simulink library "LIB_TF_G_12_StepControl"  (Simulink 8.6)
settings: Solver=ode45  StartTime=0.0  StopTime=10.0  RelTol=1e-3
PreLoadFcn:
  | if exist('tl_preloadfcn','file'), tl_preloadfcn(gcs,402); end
PostLoadFcn:
  | if exist('tl_postloadfcn','file'), tl_postloadfcn(gcs,402); end
undefined symbols (not defined in the file): ddv, u2, u3
libraries: tllib x4, LIB_TF_G_12_StepControl x1
(part 6 of 7)

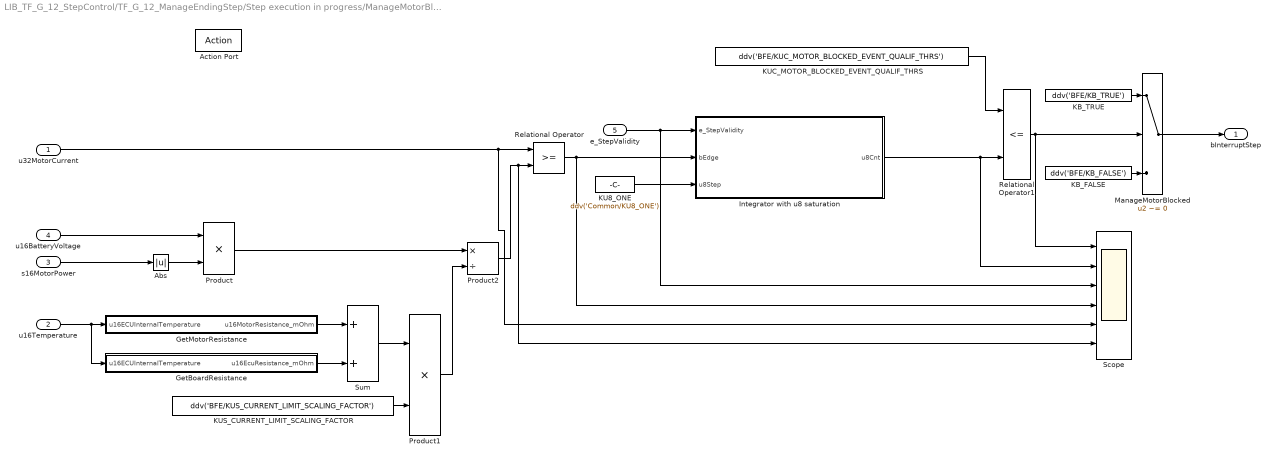
== system LIB_TF_G_12_StepControl/TF_G_12_ManageEndingStep/Step execution in progress/ManageMotorBlocked (Motor OverCurrent)/Motor Blocked Opt Activated/If Action Subsystem1 ==
  u32MotorCurrent : Inport  RequirementInfo={} %GIDa_b15262d0_e742_4384_8f9e_89978bbdea4b
  u16Temperature : Inport  RequirementInfo={} %GIDa_ef5c7aa1_d6d2_4676_bb67_ebadbb8854d8  Port=2
  s16MotorPower : Inport  RequirementInfo={} %GIDa_a7c6093a_f3fd_45c6_94cd_8623c3d3488b  Port=3
  u16BatteryVoltage : Inport  RequirementInfo={} %GIDa_ce521116_7135_4151_b5d9_8882b70060be  Port=4
  e_StepValidity : Inport  RequirementInfo={} %GIDa_ddfb933f_dae9_4570_b46d_68e419ca580a  Port=5
  Action Port : ActionPort  RequirementInfo={} %GIDa_51377548_8670_413b_8799_ae36625b9d74
  Abs : Abs  RequirementInfo={} %GIDa_8232010f_f8c2_4ccb_bbd6_00c9bee563e0  OutDataTypeStr=uint16  SaturateOnIntegerOverflow=on  mask(TL_Abs){data={'output',{'type','UInt16'},'date',735951.66847012728}}
      settings: CopyFcn=if exist('tl_reset_reviewflag','file')==2,tl_reset_reviewflag(gcbh);end  DeleteFcn=if exist('delete_tlblock','file')==2,delete_tlblock(gcbh);end  NameChangeFcn=if exist('rename_tlblock','file')==2,rename_tlblock(gcbh);end  OpenFcn=if exist('tl_open_blockdlg','file')==2,tl_open_blockdlg(gcbh);else,open_system(gcbh,'parameter');end
      mask Help: eval(['if exist(''tl_online_help'',''file'') == 2, tl_online_help(''Topic'',''TL_Abs''),else, web([''jar:file:///'',matlabroot,''/help/toolbox/simulink/help.jar!/slref/' lower(get_param(gcbh,'Blocktype')) '.html''], ''-helpbrowser''),end'])
      mask Display: plot([-0.05, 1.05, NaN, -0.05, 1.05],[.01, .01, NaN, .99, .99])
  GetBoardResistance : Subsystem  RequirementInfo={} %GIDa_d4bba72b_0433_4a1a_802a_6d5e3419819e  TreatAsAtomicUnit=on
  GetMotorResistance : Subsystem  RequirementInfo={} %GIDa_a7d90a02_c6c7_4e5e_b3b2_57b3a781c45c  TreatAsAtomicUnit=on
  Integrator with u8 saturation : Subsystem  RequirementInfo={} %GIDa_ba181890_6141_4dc0_bd10_b853b6348a4b  TreatAsAtomicUnit=on
  KB_FALSE : Constant  RequirementInfo={} %GIDa_a55cecaf_6f72_42fc_8a95_f0d92f6d4486  Value=ddv('BFE/KB_FALSE')  OutDataTypeStr=boolean  SampleTime=-1  mask(TL_Constant){data={'output',{'variable','BFE/KB_FALSE'},'date',735951.66846314818}}
      settings: CopyFcn=if exist('tl_reset_reviewflag','file')==2,tl_reset_reviewflag(gcbh);end  DeleteFcn=if exist('delete_tlblock','file')==2,delete_tlblock(gcbh);end  NameChangeFcn=if exist('rename_tlblock','file')==2,rename_tlblock(gcbh);end  OpenFcn=if exist('tl_open_blockdlg','file')==2,tl_open_blockdlg(gcbh);else,open_system(gcbh,'parameter');end
      mask Help: eval(['if exist(''tl_online_help'',''file'') == 2, tl_online_help(''Topic'',''TL_Constant''),else, web([''jar:file:///'',matlabroot,''/help/toolbox/simulink/help.jar!/slref/' lower(get_param(gcbh,'Blocktype')) '.html''], ''-helpbrowser''),end'])
      mask Display: plot([-0.05, 1.05, NaN, -0.05, 1.05],[.01, .01, NaN, .99, .99])
  KB_TRUE : Constant  RequirementInfo={} %GIDa_37d21bda_b46f_433f_b999_e144736c21a8  Value=ddv('BFE/KB_TRUE')  OutDataTypeStr=boolean  SampleTime=-1  mask(TL_Constant){data={'output',{'variable','BFE/KB_TRUE'},'date',735951.66846276622}}
      settings: CopyFcn=if exist('tl_reset_reviewflag','file')==2,tl_reset_reviewflag(gcbh);end  DeleteFcn=if exist('delete_tlblock','file')==2,delete_tlblock(gcbh);end  NameChangeFcn=if exist('rename_tlblock','file')==2,rename_tlblock(gcbh);end  OpenFcn=if exist('tl_open_blockdlg','file')==2,tl_open_blockdlg(gcbh);else,open_system(gcbh,'parameter');end
      mask Help: eval(['if exist(''tl_online_help'',''file'') == 2, tl_online_help(''Topic'',''TL_Constant''),else, web([''jar:file:///'',matlabroot,''/help/toolbox/simulink/help.jar!/slref/' lower(get_param(gcbh,'Blocktype')) '.html''], ''-helpbrowser''),end'])
      mask Display: plot([-0.05, 1.05, NaN, -0.05, 1.05],[.01, .01, NaN, .99, .99])
  KU8_ONE : Constant  RequirementInfo={} %GIDa_69ee802a_b870_416b_ab62_c046b6291559  Value=ddv('Common/KU8_ONE')  OutDataTypeStr=uint8  SampleTime=-1  mask(TL_Constant){data={'output',{'variable','Common/KU8_ONE'},'date',735951.66846239578}}
      settings: CopyFcn=if exist('tl_reset_reviewflag','file')==2,tl_reset_reviewflag(gcbh);end  DeleteFcn=if exist('delete_tlblock','file')==2,delete_tlblock(gcbh);end  NameChangeFcn=if exist('rename_tlblock','file')==2,rename_tlblock(gcbh);end  OpenFcn=if exist('tl_open_blockdlg','file')==2,tl_open_blockdlg(gcbh);else,open_system(gcbh,'parameter');end
      mask Help: eval(['if exist(''tl_online_help'',''file'') == 2, tl_online_help(''Topic'',''TL_Constant''),else, web([''jar:file:///'',matlabroot,''/help/toolbox/simulink/help.jar!/slref/' lower(get_param(gcbh,'Blocktype')) '.html''], ''-helpbrowser''),end'])
      mask Display: plot([-0.05, 1.05, NaN, -0.05, 1.05],[.01, .01, NaN, .99, .99])
  KUC_MOTOR_BLOCKED_EVENT_QUALIF_THRS : Constant  RequirementInfo={} %GIDa_b638c9ca_7e5c_4169_b0e7_1030e65cb8bd  Value=ddv('BFE/KUC_MOTOR_BLOCKED_EVENT_QUALIF_THRS')  OutDataTypeStr=uint8  SampleTime=-1  mask(TL_Constant){data={'output',{'variable','BFE/KUC_MOTOR_BLOCKED_EVENT_QUALIF_THRS'},'date',736308.64848615741}}
      settings: CopyFcn=if exist('tl_reset_reviewflag','file')==2,tl_reset_reviewflag(gcbh);end  DeleteFcn=if exist('delete_tlblock','file')==2,delete_tlblock(gcbh);end  NameChangeFcn=if exist('rename_tlblock','file')==2,rename_tlblock(gcbh);end  OpenFcn=if exist('tl_open_blockdlg','file')==2,tl_open_blockdlg(gcbh);else,open_system(gcbh,'parameter');end
      mask Help: eval(['if exist(''tl_online_help'',''file'') == 2, tl_online_help(''Topic'',''TL_Constant''),else, web([''jar:file:///'',matlabroot,''/help/toolbox/simulink/help.jar!/slref/' lower(get_param(gcbh,'Blocktype')) '.html''], ''-helpbrowser''),end'])
      mask Display: plot([-0.05, 1.05, NaN, -0.05, 1.05],[.01, .01, NaN, .99, .99])
  KUS_CURRENT_LIMIT_SCALING_FACTOR : Constant  RequirementInfo={} %GIDa_2f1f04c3_5d00_4e34_bf38_99862e862b9f  Value=ddv('BFE/KUS_CURRENT_LIMIT_SCALING_FACTOR')  OutDataTypeStr=uint16  SampleTime=-1  mask(TL_Constant){data={'output',{'variable','BFE/KUS_CURRENT_LIMIT_SCALING_FACTOR'},'date',735951.66846165515}}
      settings: CopyFcn=if exist('tl_reset_reviewflag','file')==2,tl_reset_reviewflag(gcbh);end  DeleteFcn=if exist('delete_tlblock','file')==2,delete_tlblock(gcbh);end  NameChangeFcn=if exist('rename_tlblock','file')==2,rename_tlblock(gcbh);end  OpenFcn=if exist('tl_open_blockdlg','file')==2,tl_open_blockdlg(gcbh);else,open_system(gcbh,'parameter');end
      mask Help: eval(['if exist(''tl_online_help'',''file'') == 2, tl_online_help(''Topic'',''TL_Constant''),else, web([''jar:file:///'',matlabroot,''/help/toolbox/simulink/help.jar!/slref/' lower(get_param(gcbh,'Blocktype')) '.html''], ''-helpbrowser''),end'])
      mask Display: plot([-0.05, 1.05, NaN, -0.05, 1.05],[.01, .01, NaN, .99, .99])
  ManageMotorBlocked : Switch  RequirementInfo={} %GIDa_9a329e77_4b29_4519_b45e_e6ed1365234e  Criteria=u2 ~= 0  mask(TL_Switch){data={'output',{'type','Bool'},'threshold',{'scalar',1},'date',735951.66846123838}}
      settings: CopyFcn=if exist('tl_reset_reviewflag','file')==2,tl_reset_reviewflag(gcbh);end  DeleteFcn=if exist('delete_tlblock','file')==2,delete_tlblock(gcbh);end  NameChangeFcn=if exist('rename_tlblock','file')==2,rename_tlblock(gcbh);end  OpenFcn=if exist('tl_open_blockdlg','file')==2,tl_open_blockdlg(gcbh);else,open_system(gcbh,'parameter');end
      mask Help: eval(['if exist(''tl_online_help'',''file'') == 2, tl_online_help(''Topic'',''TL_Switch''),else, web([''jar:file:///'',matlabroot,''/help/toolbox/simulink/help.jar!/slref/' lower(get_param(gcbh,'Blocktype')) '.html''], ''-helpbrowser''),end'])
      mask Display: plot([-0.05, 1.05, NaN, -0.05, 1.05],[.01, .01, NaN, .99, .99])
  Product : Product  RequirementInfo={} %GIDa_e4deacdf_ad83_4690_b51a_09e6e1684bb8  Inputs=**  OutDataTypeStr=uint32  RndMeth=Zero  mask(TL_Product){data={'output',{'type','UInt32'},'date',735951.66846074071}}
      settings: CopyFcn=if exist('tl_reset_reviewflag','file')==2,tl_reset_reviewflag(gcbh);end  DeleteFcn=if exist('delete_tlblock','file')==2,delete_tlblock(gcbh);end  NameChangeFcn=if exist('rename_tlblock','file')==2,rename_tlblock(gcbh);end  OpenFcn=if exist('tl_open_blockdlg','file')==2,tl_open_blockdlg(gcbh);else,open_system(gcbh,'parameter');end
      mask Help: eval(['if exist(''tl_online_help'',''file'') == 2, tl_online_help(''Topic'',''TL_Product''),else, web([''jar:file:///'',matlabroot,''/help/toolbox/simulink/help.jar!/slref/' lower(get_param(gcbh,'Blocktype')) '.html''], ''-helpbrowser''),end'])
      mask Display: plot([-0.05, 1.05, NaN, -0.05, 1.05],[.01, .01, NaN, .99, .99])
  Product1 : Product  RequirementInfo={} %GIDa_f39456aa_0ea8_4713_8ffb_570a378b51f3  Inputs=**  OutDataTypeStr=uint32  RndMeth=Zero  mask(TL_Product){data={'output',{'type','UInt32'},'date',735951.66846037039}}
      settings: CopyFcn=if exist('tl_reset_reviewflag','file')==2,tl_reset_reviewflag(gcbh);end  DeleteFcn=if exist('delete_tlblock','file')==2,delete_tlblock(gcbh);end  NameChangeFcn=if exist('rename_tlblock','file')==2,rename_tlblock(gcbh);end  OpenFcn=if exist('tl_open_blockdlg','file')==2,tl_open_blockdlg(gcbh);else,open_system(gcbh,'parameter');end
      mask Help: eval(['if exist(''tl_online_help'',''file'') == 2, tl_online_help(''Topic'',''TL_Product''),else, web([''jar:file:///'',matlabroot,''/help/toolbox/simulink/help.jar!/slref/' lower(get_param(gcbh,'Blocktype')) '.html''], ''-helpbrowser''),end'])
      mask Display: plot([-0.05, 1.05, NaN, -0.05, 1.05],[.01, .01, NaN, .99, .99])
  Product2 : Product  RequirementInfo={} %GIDa_a78a8f98_bcd9_4378_bd14_54184bd20a38  Inputs=*/  OutDataTypeStr=uint32  RndMeth=Zero  mask(TL_Product){data={'output',{'name','u32MaxCurrentThrs','type','UInt32'},'date',735951.66846}}
      settings: CopyFcn=if exist('tl_reset_reviewflag','file')==2,tl_reset_reviewflag(gcbh);end  DeleteFcn=if exist('delete_tlblock','file')==2,delete_tlblock(gcbh);end  NameChangeFcn=if exist('rename_tlblock','file')==2,rename_tlblock(gcbh);end  OpenFcn=if exist('tl_open_blockdlg','file')==2,tl_open_blockdlg(gcbh);else,open_system(gcbh,'parameter');end
      mask Help: eval(['if exist(''tl_online_help'',''file'') == 2, tl_online_help(''Topic'',''TL_Product''),else, web([''jar:file:///'',matlabroot,''/help/toolbox/simulink/help.jar!/slref/' lower(get_param(gcbh,'Blocktype')) '.html''], ''-helpbrowser''),end'])
      mask Display: plot([-0.05, 1.05, NaN, -0.05, 1.05],[.01, .01, NaN, .99, .99])
  Relational Operator : RelationalOperator  RequirementInfo={} %GIDa_ce1273a7_07a3_4d52_9644_bfe8f4081c88  OutDataTypeStr=boolean  mask(TL_RelationalOperator){data={'output',{'name','bMotorBlockedOccurence'},'date',735951.66845964117}}
      settings: DeleteFcn=if exist('delete_tlblock','file')==2,delete_tlblock(gcbh);end  NameChangeFcn=if exist('rename_tlblock','file')==2,rename_tlblock(gcbh);end  OpenFcn=if exist('tl_open_blockdlg','file')==2,tl_open_blockdlg(gcbh);else,open_system(gcbh,'parameter');end
      mask Help: eval(['if exist(''tl_online_help'',''file'') == 2, tl_online_help(''Topic'',''TL_RelationalOperator''),else, web([''jar:file:///'',matlabroot,''/help/toolbox/simulink/help.jar!/slref/' lower(get_param(gcbh,'Blocktype')) '.html''], ''-helpbrowser''),end'])
      mask Display: plot([-0.05, 1.05, NaN, -0.05, 1.05],[.01, .01, NaN, .99, .99])
  Relational Operator1 : RelationalOperator  RequirementInfo={} %GIDa_80bd2eb1_48b1_4a7d_aa4c_9511f66a4c53  Operator=<=  OutDataTypeStr=boolean  mask(TL_RelationalOperator){data={'date',735951.6684593634}}
      settings: DeleteFcn=if exist('delete_tlblock','file')==2,delete_tlblock(gcbh);end  NameChangeFcn=if exist('rename_tlblock','file')==2,rename_tlblock(gcbh);end  OpenFcn=if exist('tl_open_blockdlg','file')==2,tl_open_blockdlg(gcbh);else,open_system(gcbh,'parameter');end
      mask Help: eval(['if exist(''tl_online_help'',''file'') == 2, tl_online_help(''Topic'',''TL_RelationalOperator''),else, web([''jar:file:///'',matlabroot,''/help/toolbox/simulink/help.jar!/slref/' lower(get_param(gcbh,'Blocktype')) '.html''], ''-helpbrowser''),end'])
      mask Display: plot([-0.05, 1.05, NaN, -0.05, 1.05],[.01, .01, NaN, .99, .99])
  Scope : Scope  NumInputPorts=6
  Sum : Sum  RequirementInfo={} %GIDa_eb212244_389f_4475_89c7_cc1c19e88d30  OutDataTypeStr=uint16  mask(TL_Sum){data={'output',{'name','u16ResistEquiv','type','UInt16'},'date',735951.66845909727}}
      settings: CopyFcn=if exist('tl_reset_reviewflag','file')==2,tl_reset_reviewflag(gcbh);end  DeleteFcn=if exist('delete_tlblock','file')==2,delete_tlblock(gcbh);end  NameChangeFcn=if exist('rename_tlblock','file')==2,rename_tlblock(gcbh);end  OpenFcn=if exist('tl_open_blockdlg','file')==2,tl_open_blockdlg(gcbh);else,open_system(gcbh,'parameter');end
      mask Help: eval(['if exist(''tl_online_help'',''file'') == 2, tl_online_help(''Topic'',''TL_Sum''),else, web([''jar:file:///'',matlabroot,''/help/toolbox/simulink/help.jar!/slref/' lower(get_param(gcbh,'Blocktype')) '.html''], ''-helpbrowser''),end'])
      mask Display: plot([-0.05, 1.05, NaN, -0.05, 1.05],[.01, .01, NaN, .99, .99])
  bInterruptStep : Outport  RequirementInfo={} %GIDa_411d1535_bc35_4078_b831_458384912e14
  wires:
  s16MotorPower/1 -> Abs/1
  Abs/1 -> Product/2
  u16BatteryVoltage/1 -> Product/1
  Product/1 -> Product2/1
  KUS_CURRENT_LIMIT_SCALING_FACTOR/1 -> Product1/2
  u16Temperature/1 -> GetMotorResistance/1(u16ECUInternalTemperature), GetBoardResistance/1(u16ECUInternalTemperature)
  GetMotorResistance/1(u16MotorResistance_mOhm) -> Sum/1
  GetBoardResistance/1(u16EcuResistance_mOhm) -> Sum/2
  u32MotorCurrent/1 -> Relational Operator/1, Scope/5
  Product2/1 -> Relational Operator/2, Scope/6
  Relational Operator/1 -> Scope/4, Integrator with u8 saturation/2(bEdge)
  ManageMotorBlocked/1 -> bInterruptStep/1
  KB_FALSE/1 -> ManageMotorBlocked/3
  KUC_MOTOR_BLOCKED_EVENT_QUALIF_THRS/1 -> Relational Operator1/1
  Integrator with u8 saturation/1(u8Cnt) -> Scope/2, Relational Operator1/2
  Relational Operator1/1 -> Scope/1, ManageMotorBlocked/2
  KB_TRUE/1 -> ManageMotorBlocked/1
  KU8_ONE/1 -> Integrator with u8 saturation/3(u8Step)
  Sum/1 -> Product1/1
  Product1/1 -> Product2/2
  e_StepValidity/1 -> Scope/3, Integrator with u8 saturation/1(e_StepValidity)

== system LIB_TF_G_12_StepControl/TF_G_12_ControlStepExecution/New Step started/Adapt Step Target Value/Temperature Weighted/Step Order Positive/Switch Case Action Subsystem ==
  In1 : Inport
  Action Port : ActionPort
  SelectTens0Factor : Lookup_n-D  RequirementInfo={} %GIDa_30e6e979_46d8_46e5_be26_3ce3c57d4d52  NumberOfTableDimensions=1  BreakpointsForDimension1=ddv('BFE_Config_Data/CFG_au16TempWeightIndexTens0')  BreakpointsForDimension2=[1:3]  IndexSearchMethod=Linear search  Table=ddv('BFE_Config_Data/CFG_au8TempWeightFactorsTens0')  ExtrapMethod=Clip  OutDataTypeStr=uint8  InputSameDT=on  mask(TL_Lookup1D){data={'input',{'variable','BFE_Config_Data/CFG_au16TempWeightIndexTens0'},'output',{'type','UInt8'},'table',{'variable','BFE_Config_Data/CFG_au8TempWeightFactorsTens0'},'date',735951.66798973375}}
      settings: CopyFcn=if exist('tl_reset_reviewflag','file')==2,tl_reset_reviewflag(gcbh);end  DeleteFcn=if exist('delete_tlblock','file')==2,delete_tlblock(gcbh);end  NameChangeFcn=if exist('rename_tlblock','file')==2,rename_tlblock(gcbh);end  OpenFcn=if exist('tl_open_blockdlg','file')==2,tl_open_blockdlg(gcbh);else,open_system(gcbh,'parameter');end
      mask Help: eval(['if exist(''tl_online_help'',''file'') == 2, tl_online_help(''Topic'',''TL_Lookup1D''),else, web([''jar:file:///'',matlabroot,''/help/toolbox/simulink/help.jar!/slref/' lower(get_param(gcbh,'Blocktype')) '.html''], ''-helpbrowser''),end'])
      mask Display: plot([-0.05, 1.05, NaN, -0.05, 1.05],[.01, .01, NaN, .99, .99])
  Out1 : Outport  InitialOutput=64
  wires:
  In1/1 -> SelectTens0Factor/1
  SelectTens0Factor/1 -> Out1/1

== system LIB_TF_G_12_StepControl/TF_G_12_ControlStepExecution/New Step started/Adapt Step Target Value/Temperature Weighted/Step Order Positive/Switch Case Action Subsystem1 ==
  In1 : Inport
  Action Port : ActionPort
  SelectTens1Factor : Lookup_n-D  RequirementInfo={} %GIDa_6ab403d0_ae2f_49a7_8709_c8e90e2e10f4  NumberOfTableDimensions=1  BreakpointsForDimension1=ddv('BFE_Config_Data/CFG_au16TempWeightIndexTens1')  BreakpointsForDimension2=[1:3]  IndexSearchMethod=Linear search  Table=ddv('BFE_Config_Data/CFG_au8TempWeightFactorsTens1')  ExtrapMethod=Clip  OutDataTypeStr=uint8  InputSameDT=on  mask(TL_Lookup1D){data={'input',{'variable','BFE_Config_Data/CFG_au16TempWeightIndexTens1'},'output',{'type','UInt8'},'table',{'variable','BFE_Config_Data/CFG_au8TempWeightFactorsTens1'},'date',735951.66798855329}}
      settings: CopyFcn=if exist('tl_reset_reviewflag','file')==2,tl_reset_reviewflag(gcbh);end  DeleteFcn=if exist('delete_tlblock','file')==2,delete_tlblock(gcbh);end  NameChangeFcn=if exist('rename_tlblock','file')==2,rename_tlblock(gcbh);end  OpenFcn=if exist('tl_open_blockdlg','file')==2,tl_open_blockdlg(gcbh);else,open_system(gcbh,'parameter');end
      mask Help: eval(['if exist(''tl_online_help'',''file'') == 2, tl_online_help(''Topic'',''TL_Lookup1D''),else, web([''jar:file:///'',matlabroot,''/help/toolbox/simulink/help.jar!/slref/' lower(get_param(gcbh,'Blocktype')) '.html''], ''-helpbrowser''),end'])
      mask Display: plot([-0.05, 1.05, NaN, -0.05, 1.05],[.01, .01, NaN, .99, .99])
  Out1 : Outport  InitialOutput=64
  wires:
  In1/1 -> SelectTens1Factor/1
  SelectTens1Factor/1 -> Out1/1

== system LIB_TF_G_12_StepControl/TF_G_12_ControlStepExecution/New Step started/Adapt Step Target Value/Temperature Weighted/Step Order Positive/Switch Case Action Subsystem2 ==
  In1 : Inport
  Action Port : ActionPort
  SelectTens0Factor : Lookup_n-D  RequirementInfo={} %GIDa_a49215d2_5d52_4dd0_93bc_76a4194c5446  NumberOfTableDimensions=1  BreakpointsForDimension1=ddv('BFE_Config_Data/CFG_au16TempWeightIndexTens2')  BreakpointsForDimension2=[1:3]  IndexSearchMethod=Linear search  Table=ddv('BFE_Config_Data/CFG_au8TempWeightFactorsTens2')  ExtrapMethod=Clip  OutDataTypeStr=uint8  InputSameDT=on  mask(TL_Lookup1D){data={'input',{'variable','BFE_Config_Data/CFG_au16TempWeightIndexTens2'},'output',{'type','UInt8'},'table',{'variable','BFE_Config_Data/CFG_au8TempWeightFactorsTens2'},'date',735951.66798738425}}
      settings: CopyFcn=if exist('tl_reset_reviewflag','file')==2,tl_reset_reviewflag(gcbh);end  DeleteFcn=if exist('delete_tlblock','file')==2,delete_tlblock(gcbh);end  NameChangeFcn=if exist('rename_tlblock','file')==2,rename_tlblock(gcbh);end  OpenFcn=if exist('tl_open_blockdlg','file')==2,tl_open_blockdlg(gcbh);else,open_system(gcbh,'parameter');end
      mask Help: eval(['if exist(''tl_online_help'',''file'') == 2, tl_online_help(''Topic'',''TL_Lookup1D''),else, web([''jar:file:///'',matlabroot,''/help/toolbox/simulink/help.jar!/slref/' lower(get_param(gcbh,'Blocktype')) '.html''], ''-helpbrowser''),end'])
      mask Display: plot([-0.05, 1.05, NaN, -0.05, 1.05],[.01, .01, NaN, .99, .99])
  Out1 : Outport  InitialOutput=64
  wires:
  In1/1 -> SelectTens0Factor/1
  SelectTens0Factor/1 -> Out1/1

== system LIB_TF_G_12_StepControl/TF_G_12_ControlStepExecution/New Step started/Adapt Step Target Value/Temperature Weighted/Step Order Positive/Switch Case Action Subsystem3 ==
  In1 : Inport
  Action Port : ActionPort
  SelectTens3Factor : Lookup_n-D  RequirementInfo={} %GIDa_829bd617_24c4_4656_b5fe_8018b3a5d423  NumberOfTableDimensions=1  BreakpointsForDimension1=ddv('BFE_Config_Data/CFG_au16TempWeightIndexTens3')  BreakpointsForDimension2=[1:3]  IndexSearchMethod=Linear search  Table=ddv('BFE_Config_Data/CFG_au8TempWeightFactorsTens3')  ExtrapMethod=Clip  OutDataTypeStr=uint8  InputSameDT=on  mask(TL_Lookup1D){data={'input',{'variable','BFE_Config_Data/CFG_au16TempWeightIndexTens3'},'output',{'type','UInt8'},'table',{'variable','BFE_Config_Data/CFG_au8TempWeightFactorsTens3'},'date',735951.66798612266}}
      settings: CopyFcn=if exist('tl_reset_reviewflag','file')==2,tl_reset_reviewflag(gcbh);end  DeleteFcn=if exist('delete_tlblock','file')==2,delete_tlblock(gcbh);end  NameChangeFcn=if exist('rename_tlblock','file')==2,rename_tlblock(gcbh);end  OpenFcn=if exist('tl_open_blockdlg','file')==2,tl_open_blockdlg(gcbh);else,open_system(gcbh,'parameter');end
      mask Help: eval(['if exist(''tl_online_help'',''file'') == 2, tl_online_help(''Topic'',''TL_Lookup1D''),else, web([''jar:file:///'',matlabroot,''/help/toolbox/simulink/help.jar!/slref/' lower(get_param(gcbh,'Blocktype')) '.html''], ''-helpbrowser''),end'])
      mask Display: plot([-0.05, 1.05, NaN, -0.05, 1.05],[.01, .01, NaN, .99, .99])
  Out1 : Outport  InitialOutput=64
  wires:
  In1/1 -> SelectTens3Factor/1
  SelectTens3Factor/1 -> Out1/1

== system LIB_TF_G_12_StepControl/TF_G_12_ControlStepExecution/New Step started/Adapt Step Target Value/Temperature Weighted/Step Order Positive/Switch Case Action Subsystem4 ==
  Action Port : ActionPort
  KU8_NO_WEIGHT : Constant  RequirementInfo={} %GIDa_ff5d2a09_23d1_4d0b_a7dd_e6af86c1e003  Value=ddv('BFE/KUC_NEUTRAL_WEIGHT')  OutDataTypeStr=uint8  mask(TL_Constant){data={'output',{'variable','BFE/KUC_NEUTRAL_WEIGHT'},'date',735951.66798501159}}
      settings: CopyFcn=if exist('tl_reset_reviewflag','file')==2,tl_reset_reviewflag(gcbh);end  DeleteFcn=if exist('delete_tlblock','file')==2,delete_tlblock(gcbh);end  NameChangeFcn=if exist('rename_tlblock','file')==2,rename_tlblock(gcbh);end  OpenFcn=if exist('tl_open_blockdlg','file')==2,tl_open_blockdlg(gcbh);else,open_system(gcbh,'parameter');end
      mask Help: eval(['if exist(''tl_online_help'',''file'') == 2, tl_online_help(''Topic'',''TL_Constant''),else, web([''jar:file:///'',matlabroot,''/help/toolbox/simulink/help.jar!/slref/' lower(get_param(gcbh,'Blocktype')) '.html''], ''-helpbrowser''),end'])
      mask Display: plot([-0.05, 1.05, NaN, -0.05, 1.05],[.01, .01, NaN, .99, .99])
  Out1 : Outport  InitialOutput=64
  wires:
  KU8_NO_WEIGHT/1 -> Out1/1

== system LIB_TF_G_12_StepControl/TF_G_12_ControlStepExecution/New Step started/AdaptOrderType/If Action Subsystem/If Action Subsystem/If Action Subsystem ==
  Action Port : ActionPort
  KU8_HIGH_POWER_STEP_TYPE : Constant  RequirementInfo={} %GIDa_df847f2a_2e24_49ac_ba18_0acb59fe60e5  Value=ddv('BFE/Step_Def/KU8_HIGH_POWER_STEP_TYPE')  OutDataTypeStr=uint8  mask(TL_Constant){data={'output',{'variable','BFE/Step_Def/KU8_HIGH_POWER_STEP_TYPE'},'date',735951.66798312496}}
      settings: CopyFcn=if exist('tl_reset_reviewflag','file')==2,tl_reset_reviewflag(gcbh);end  DeleteFcn=if exist('delete_tlblock','file')==2,delete_tlblock(gcbh);end  NameChangeFcn=if exist('rename_tlblock','file')==2,rename_tlblock(gcbh);end  OpenFcn=if exist('tl_open_blockdlg','file')==2,tl_open_blockdlg(gcbh);else,open_system(gcbh,'parameter');end
      mask Help: eval(['if exist(''tl_online_help'',''file'') == 2, tl_online_help(''Topic'',''TL_Constant''),else, web([''jar:file:///'',matlabroot,''/help/toolbox/simulink/help.jar!/slref/' lower(get_param(gcbh,'Blocktype')) '.html''], ''-helpbrowser''),end'])
      mask Display: plot([-0.05, 1.05, NaN, -0.05, 1.05],[.01, .01, NaN, .99, .99])
  Out1 : Outport  RequirementInfo={} %GIDa_99f22b95_c8dd_4676_b0e9_280696c48473  InitialOutput=65
  wires:
  KU8_HIGH_POWER_STEP_TYPE/1 -> Out1/1

== system LIB_TF_G_12_StepControl/TF_G_12_ControlStepExecution/New Step started/AdaptOrderType/If Action Subsystem/If Action Subsystem/If Action Subsystem1 ==
  Action Port : ActionPort
  KU8_CURRENT_STEP_TYPE : Constant  RequirementInfo={} %GIDa_d9a6b188_624e_4afe_9257_f56dd6fd5805  Value=ddv('BFE/Step_Def/KU8_CURRENT_STEP_TYPE')  OutDataTypeStr=uint8  mask(TL_Constant){data={'output',{'variable','BFE/Step_Def/KU8_CURRENT_STEP_TYPE'},'date',735951.66798274301}}
      settings: CopyFcn=if exist('tl_reset_reviewflag','file')==2,tl_reset_reviewflag(gcbh);end  DeleteFcn=if exist('delete_tlblock','file')==2,delete_tlblock(gcbh);end  NameChangeFcn=if exist('rename_tlblock','file')==2,rename_tlblock(gcbh);end  OpenFcn=if exist('tl_open_blockdlg','file')==2,tl_open_blockdlg(gcbh);else,open_system(gcbh,'parameter');end
      mask Help: eval(['if exist(''tl_online_help'',''file'') == 2, tl_online_help(''Topic'',''TL_Constant''),else, web([''jar:file:///'',matlabroot,''/help/toolbox/simulink/help.jar!/slref/' lower(get_param(gcbh,'Blocktype')) '.html''], ''-helpbrowser''),end'])
      mask Display: plot([-0.05, 1.05, NaN, -0.05, 1.05],[.01, .01, NaN, .99, .99])
  Out1 : Outport  RequirementInfo={} %GIDa_7626f397_348f_4ddb_b76c_b204b88fff44  InitialOutput=1
  wires:
  KU8_CURRENT_STEP_TYPE/1 -> Out1/1

== system LIB_TF_G_12_StepControl/TF_G_12_ControlStepExecution/New Step started/AdaptOrderType/If Action Subsystem/If Action Subsystem1/If Action Subsystem ==
  Action Port : ActionPort
  KU8_PID_MOTOR_STEP_TYPE : Constant  RequirementInfo={} %GIDa_e142d0e1_c548_48b2_921b_2fe3b8470026  Value=ddv('BFE/Step_Def/KU8_PID_MOTOR_STEP_TYPE')  OutDataTypeStr=uint8  mask(TL_Constant){data={'output',{'variable','BFE/Step_Def/KU8_PID_MOTOR_STEP_TYPE'},'date',735951.66798182868}}
      settings: CopyFcn=if exist('tl_reset_reviewflag','file')==2,tl_reset_reviewflag(gcbh);end  DeleteFcn=if exist('delete_tlblock','file')==2,delete_tlblock(gcbh);end  NameChangeFcn=if exist('rename_tlblock','file')==2,rename_tlblock(gcbh);end  OpenFcn=if exist('tl_open_blockdlg','file')==2,tl_open_blockdlg(gcbh);else,open_system(gcbh,'parameter');end
      mask Help: eval(['if exist(''tl_online_help'',''file'') == 2, tl_online_help(''Topic'',''TL_Constant''),else, web([''jar:file:///'',matlabroot,''/help/toolbox/simulink/help.jar!/slref/' lower(get_param(gcbh,'Blocktype')) '.html''], ''-helpbrowser''),end'])
      mask Display: plot([-0.05, 1.05, NaN, -0.05, 1.05],[.01, .01, NaN, .99, .99])
  Out1 : Outport  RequirementInfo={} %GIDa_1e4f8453_dbbb_4979_84a0_58694600bcee  InitialOutput=33
  wires:
  KU8_PID_MOTOR_STEP_TYPE/1 -> Out1/1

== system LIB_TF_G_12_StepControl/TF_G_12_ControlStepExecution/New Step started/AdaptOrderType/If Action Subsystem/If Action Subsystem1/If Action Subsystem1 ==
  Action Port : ActionPort
  KU8_CURRENT_STEP_TYPE : Constant  RequirementInfo={} %GIDa_3781a4fc_ae23_4550_8bfa_0c78be6a4672  Value=ddv('BFE/Step_Def/KU8_CURRENT_STEP_TYPE')  OutDataTypeStr=uint8  mask(TL_Constant){data={'output',{'variable','BFE/Step_Def/KU8_CURRENT_STEP_TYPE'},'date',735951.66798145836}}
      settings: CopyFcn=if exist('tl_reset_reviewflag','file')==2,tl_reset_reviewflag(gcbh);end  DeleteFcn=if exist('delete_tlblock','file')==2,delete_tlblock(gcbh);end  NameChangeFcn=if exist('rename_tlblock','file')==2,rename_tlblock(gcbh);end  OpenFcn=if exist('tl_open_blockdlg','file')==2,tl_open_blockdlg(gcbh);else,open_system(gcbh,'parameter');end
      mask Help: eval(['if exist(''tl_online_help'',''file'') == 2, tl_online_help(''Topic'',''TL_Constant''),else, web([''jar:file:///'',matlabroot,''/help/toolbox/simulink/help.jar!/slref/' lower(get_param(gcbh,'Blocktype')) '.html''], ''-helpbrowser''),end'])
      mask Display: plot([-0.05, 1.05, NaN, -0.05, 1.05],[.01, .01, NaN, .99, .99])
  Out1 : Outport  RequirementInfo={} %GIDa_c15a2872_8ee5_4a8e_ab1f_535dcec18674  InitialOutput=1
  wires:
  KU8_CURRENT_STEP_TYPE/1 -> Out1/1

== system LIB_TF_G_12_StepControl/TF_G_12_ControlStepExecution/New Step started/AdaptOrderType/If Action Subsystem/If Action Subsystem2/If Action Subsystem ==
  Action Port : ActionPort
  KU8_PID_SUPPLY_STEP_TYPE : Constant  RequirementInfo={} %GIDa_921c2e55_3675_4919_b837_bc442b5dd5e8  Value=ddv('BFE/Step_Def/KU8_PID_SUPPLY_STEP_TYPE')  OutDataTypeStr=uint8  mask(TL_Constant){data={'output',{'variable','BFE/Step_Def/KU8_PID_SUPPLY_STEP_TYPE'},'date',735951.66798021994}}
      settings: CopyFcn=if exist('tl_reset_reviewflag','file')==2,tl_reset_reviewflag(gcbh);end  DeleteFcn=if exist('delete_tlblock','file')==2,delete_tlblock(gcbh);end  NameChangeFcn=if exist('rename_tlblock','file')==2,rename_tlblock(gcbh);end  OpenFcn=if exist('tl_open_blockdlg','file')==2,tl_open_blockdlg(gcbh);else,open_system(gcbh,'parameter');end
      mask Help: eval(['if exist(''tl_online_help'',''file'') == 2, tl_online_help(''Topic'',''TL_Constant''),else, web([''jar:file:///'',matlabroot,''/help/toolbox/simulink/help.jar!/slref/' lower(get_param(gcbh,'Blocktype')) '.html''], ''-helpbrowser''),end'])
      mask Display: plot([-0.05, 1.05, NaN, -0.05, 1.05],[.01, .01, NaN, .99, .99])
  Out1 : Outport  RequirementInfo={} %GIDa_08342348_1362_4bab_bcdd_c80edb7eea99  InitialOutput=17
  wires:
  KU8_PID_SUPPLY_STEP_TYPE/1 -> Out1/1

== system LIB_TF_G_12_StepControl/TF_G_12_ControlStepExecution/New Step started/AdaptOrderType/If Action Subsystem/If Action Subsystem2/If Action Subsystem1 ==
  Action Port : ActionPort
  KU8_CURRENT_STEP_TYPE : Constant  RequirementInfo={} %GIDa_83b9c031_1818_4e6e_b01f_7b63621e5298  Value=ddv('BFE/Step_Def/KU8_CURRENT_STEP_TYPE')  OutDataTypeStr=uint8  mask(TL_Constant){data={'output',{'variable','BFE/Step_Def/KU8_CURRENT_STEP_TYPE'},'date',735951.6679798495}}
      settings: CopyFcn=if exist('tl_reset_reviewflag','file')==2,tl_reset_reviewflag(gcbh);end  DeleteFcn=if exist('delete_tlblock','file')==2,delete_tlblock(gcbh);end  NameChangeFcn=if exist('rename_tlblock','file')==2,rename_tlblock(gcbh);end  OpenFcn=if exist('tl_open_blockdlg','file')==2,tl_open_blockdlg(gcbh);else,open_system(gcbh,'parameter');end
      mask Help: eval(['if exist(''tl_online_help'',''file'') == 2, tl_online_help(''Topic'',''TL_Constant''),else, web([''jar:file:///'',matlabroot,''/help/toolbox/simulink/help.jar!/slref/' lower(get_param(gcbh,'Blocktype')) '.html''], ''-helpbrowser''),end'])
      mask Display: plot([-0.05, 1.05, NaN, -0.05, 1.05],[.01, .01, NaN, .99, .99])
  Out1 : Outport  RequirementInfo={} %GIDa_cbabd11e_394e_47bf_a014_96fb7079dc6a  InitialOutput=1
  wires:
  KU8_CURRENT_STEP_TYPE/1 -> Out1/1

== system LIB_TF_G_12_StepControl/TF_G_12_ManageEndingStep/Step execution in progress/ManageMotorBlocked (Motor OverCurrent)/Motor Blocked Opt Activated/If Action Subsystem1/GetBoardResistance ==
  u16ECUInternalTemperature : Inport  RequirementInfo={} %GIDa_560f37dd_7a65_4551_b6e5_2f94777ba277  PortDimensions=1  mask(TL_Inport){data={'output',{'type','UInt16'},'autosar',{'useautosarcommunication',1,'kind',5,'operationargument','AUTOLIV/GlobalDictionary/ClientServerInterfaces/icsResistance/Operations/Get/OperationArguments/u16ECUInternalTemperature'},'date',736467.66186133097}}
      settings: CopyFcn=if exist('tl_reset_reviewflag','file')==2,tl_reset_reviewflag(gcbh);end  DeleteFcn=if exist('delete_tlblock','file')==2,delete_tlblock(gcbh);end  NameChangeFcn=if exist('rename_tlblock','file')==2,rename_tlblock(gcbh);end  OpenFcn=if exist('tl_open_blockdlg','file')==2,tl_open_blockdlg(gcbh);else,open_system(gcbh,'parameter');end
      mask Help: eval(['if exist(''tl_online_help'',''file'') == 2, tl_online_help(''Topic'',''TL_Inport''),else, web([''jar:file:///'',matlabroot,''/help/toolbox/simulink/help.jar!/slref/' lower(get_param(gcbh,'Blocktype')) '.html''], ''-helpbrowser''),end'])
      mask Display: plot([0.2 0.35 NaN 0.65 0.8],[0 1 NaN 0 1]);
  Function : tllib/Function  data={'autosar',{'useautosarspecification',1,'functionrole',3,'clientport','pclECU_R','operation','Get','clientsoftwarecomponent','SwComponentType/BFE_AC_BeltFunctionExecution'},'date',736809.44007498841}  displayString=|
      | OPERATION CALL
      | (SYNCHRONOUS)
  Terminator : Terminator
  u16NvmECUResistance : Constant  RequirementInfo={} %GIDa_228fb5c7_d658_4bdc_91e0_b698bba073d1  Value=ddv('BFE_Config_Data/CFG_u16EcuResistance')  OutDataTypeStr=uint16  SampleTime=-1  mask(TL_Constant){data={'output',{'variable','BFE_Config_Data/CFG_u16EcuResistance'},'date',735951.66846902773}}
      settings: CopyFcn=if exist('tl_reset_reviewflag','file')==2,tl_reset_reviewflag(gcbh);end  DeleteFcn=if exist('delete_tlblock','file')==2,delete_tlblock(gcbh);end  NameChangeFcn=if exist('rename_tlblock','file')==2,rename_tlblock(gcbh);end  OpenFcn=if exist('tl_open_blockdlg','file')==2,tl_open_blockdlg(gcbh);else,open_system(gcbh,'parameter');end
      mask Help: eval(['if exist(''tl_online_help'',''file'') == 2, tl_online_help(''Topic'',''TL_Constant''),else, web([''jar:file:///'',matlabroot,''/help/toolbox/simulink/help.jar!/slref/' lower(get_param(gcbh,'Blocktype')) '.html''], ''-helpbrowser''),end'])
      mask Display: plot([-0.05, 1.05, NaN, -0.05, 1.05],[.01, .01, NaN, .99, .99])
  u16EcuResistance_mOhm : Outport  RequirementInfo={} %GIDa_ec6415b5_1690_4e8d_b9a3_9b02705e5f30  PortDimensions=1  mask(TL_Outport){data={'autosar',{'useautosarcommunication',1,'kind',5,'operationargument','AUTOLIV/GlobalDictionary/ClientServerInterfaces/icsResistance/Operations/Get/OperationArguments/pu16Resistance_mOhm'},'date',736467.66198516206}}
      settings: CopyFcn=if exist('tl_reset_reviewflag','file')==2,tl_reset_reviewflag(gcbh);end  DeleteFcn=if exist('delete_tlblock','file')==2,delete_tlblock(gcbh);end  NameChangeFcn=if exist('rename_tlblock','file')==2,rename_tlblock(gcbh);end  OpenFcn=if exist('tl_open_blockdlg','file')==2,tl_open_blockdlg(gcbh);else,open_system(gcbh,'parameter');end
      mask Help: eval(['if exist(''tl_online_help'',''file'') == 2, tl_online_help(''Topic'',''TL_Outport''),else, web([''jar:file:///'',matlabroot,''/help/toolbox/simulink/help.jar!/slref/' lower(get_param(gcbh,'Blocktype')) '.html''], ''-helpbrowser''),end'])
      mask Display: plot([0.2 0.35 NaN 0.65 0.8],[0 1 NaN 0 1]);
  wires:
  u16NvmECUResistance/1 -> u16EcuResistance_mOhm/1
  u16ECUInternalTemperature/1 -> Terminator/1

== system LIB_TF_G_12_StepControl/TF_G_12_ManageEndingStep/Step execution in progress/ManageMotorBlocked (Motor OverCurrent)/Motor Blocked Opt Activated/If Action Subsystem1/GetMotorResistance ==
  u16ECUInternalTemperature : Inport  RequirementInfo={} %GIDa_060a0bd5_47f2_40de_ab8c_cce0cbc868fc  PortDimensions=1  mask(TL_Inport){data={'output',{'type','UInt16'},'autosar',{'useautosarcommunication',1,'kind',5,'operationargument','AUTOLIV/GlobalDictionary/ClientServerInterfaces/icsResistance/Operations/Get/OperationArguments/u16ECUInternalTemperature'},'date',736467.66143432865}}
      settings: CopyFcn=if exist('tl_reset_reviewflag','file')==2,tl_reset_reviewflag(gcbh);end  DeleteFcn=if exist('delete_tlblock','file')==2,delete_tlblock(gcbh);end  NameChangeFcn=if exist('rename_tlblock','file')==2,rename_tlblock(gcbh);end  OpenFcn=if exist('tl_open_blockdlg','file')==2,tl_open_blockdlg(gcbh);else,open_system(gcbh,'parameter');end
      mask Help: eval(['if exist(''tl_online_help'',''file'') == 2, tl_online_help(''Topic'',''TL_Inport''),else, web([''jar:file:///'',matlabroot,''/help/toolbox/simulink/help.jar!/slref/' lower(get_param(gcbh,'Blocktype')) '.html''], ''-helpbrowser''),end'])
      mask Display: plot([0.2 0.35 NaN 0.65 0.8],[0 1 NaN 0 1]);
  Function : tllib/Function  data={'autosar',{'useautosarspecification',1,'functionrole',3,'clientport','pclMotor_R','operation','Get','clientsoftwarecomponent','SwComponentType/BFE_AC_BeltFunctionExecution'},'date',736809.44007614581}  displayString=|
      | OPERATION CALL
      | (SYNCHRONOUS)
  Terminator : Terminator
  u16NvmMotorResistance : Constant  RequirementInfo={} %GIDa_9e7b358b_f8ae_4f14_b8a3_6cc0eeab9745  Value=ddv('BFE_Config_Data/CFG_u16MotorResistance')  OutDataTypeStr=uint16  SampleTime=-1  mask(TL_Constant){data={'output',{'variable','BFE_Config_Data/CFG_u16MotorResistance'},'date',735951.66846710653}}
      settings: CopyFcn=if exist('tl_reset_reviewflag','file')==2,tl_reset_reviewflag(gcbh);end  DeleteFcn=if exist('delete_tlblock','file')==2,delete_tlblock(gcbh);end  NameChangeFcn=if exist('rename_tlblock','file')==2,rename_tlblock(gcbh);end  OpenFcn=if exist('tl_open_blockdlg','file')==2,tl_open_blockdlg(gcbh);else,open_system(gcbh,'parameter');end
      mask Help: eval(['if exist(''tl_online_help'',''file'') == 2, tl_online_help(''Topic'',''TL_Constant''),else, web([''jar:file:///'',matlabroot,''/help/toolbox/simulink/help.jar!/slref/' lower(get_param(gcbh,'Blocktype')) '.html''], ''-helpbrowser''),end'])
      mask Display: plot([-0.05, 1.05, NaN, -0.05, 1.05],[.01, .01, NaN, .99, .99])
  u16MotorResistance_mOhm : Outport  RequirementInfo={} %GIDa_e599d12b_3eaf_427a_8456_9596e6a35667  PortDimensions=1  mask(TL_Outport){data={'autosar',{'useautosarcommunication',1,'kind',5,'operationargument','AUTOLIV/GlobalDictionary/ClientServerInterfaces/icsResistance/Operations/Get/OperationArguments/pu16Resistance_mOhm'},'date',736467.66161453701}}
      settings: CopyFcn=if exist('tl_reset_reviewflag','file')==2,tl_reset_reviewflag(gcbh);end  DeleteFcn=if exist('delete_tlblock','file')==2,delete_tlblock(gcbh);end  NameChangeFcn=if exist('rename_tlblock','file')==2,rename_tlblock(gcbh);end  OpenFcn=if exist('tl_open_blockdlg','file')==2,tl_open_blockdlg(gcbh);else,open_system(gcbh,'parameter');end
      mask Help: eval(['if exist(''tl_online_help'',''file'') == 2, tl_online_help(''Topic'',''TL_Outport''),else, web([''jar:file:///'',matlabroot,''/help/toolbox/simulink/help.jar!/slref/' lower(get_param(gcbh,'Blocktype')) '.html''], ''-helpbrowser''),end'])
      mask Display: plot([0.2 0.35 NaN 0.65 0.8],[0 1 NaN 0 1]);
  wires:
  u16ECUInternalTemperature/1 -> Terminator/1
  u16NvmMotorResistance/1 -> u16MotorResistance_mOhm/1

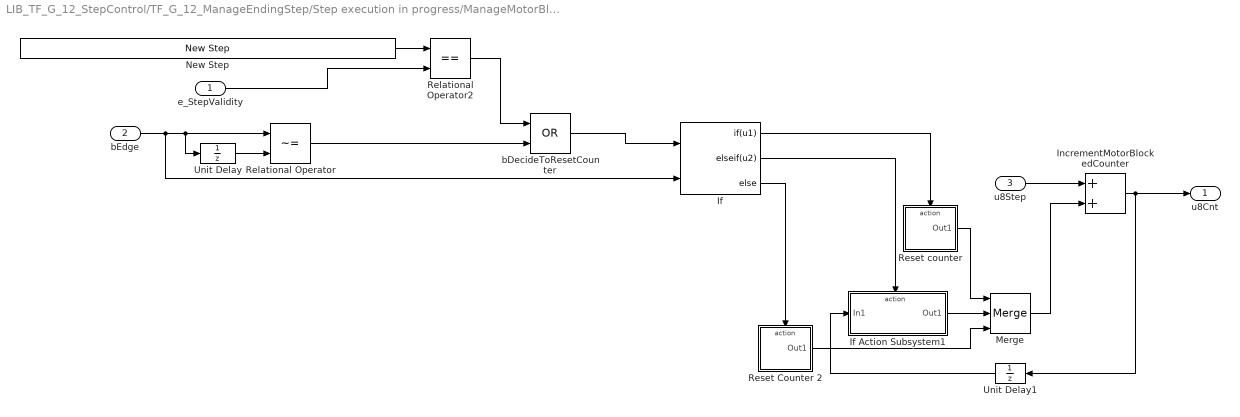
== system LIB_TF_G_12_StepControl/TF_G_12_ManageEndingStep/Step execution in progress/ManageMotorBlocked (Motor OverCurrent)/Motor Blocked Opt Activated/If Action Subsystem1/Integrator with u8 saturation ==
  e_StepValidity : Inport
  bEdge : Inport  RequirementInfo={} %GIDa_e3bbb62d_9c17_43c8_85dc_e2ba79688d74  Port=2
  u8Step : Inport  RequirementInfo={} %GIDa_b3d16149_9d67_4469_8fa7_f023b33af4f6  Port=3
  If : If  RequirementInfo={} %GIDa_bba06898_e575_44cf_b0e9_1878577792fa  NumInputs=2  IfExpression=u1  ElseIfExpressions=u2
  If Action Subsystem1 : Subsystem  RequirementInfo={} %GIDa_a5a0ec77_59af_4aff_9080_09e583e7c648  TreatAsAtomicUnit=on
  IncrementMotorBlockedCounter : Sum  RequirementInfo={} %GIDa_8f54d325_7614_408a_aab0_b50619656801  OutDataTypeStr=uint8  SaturateOnIntegerOverflow=on  mask(TL_Sum){data={'output',{'name','u8MotorBlockedCnt','type','UInt8','checkmin',1,'checkmax',1},'date',735951.66846454865}}
      settings: CopyFcn=if exist('tl_reset_reviewflag','file')==2,tl_reset_reviewflag(gcbh);end  DeleteFcn=if exist('delete_tlblock','file')==2,delete_tlblock(gcbh);end  NameChangeFcn=if exist('rename_tlblock','file')==2,rename_tlblock(gcbh);end  OpenFcn=if exist('tl_open_blockdlg','file')==2,tl_open_blockdlg(gcbh);else,open_system(gcbh,'parameter');end
      mask Help: eval(['if exist(''tl_online_help'',''file'') == 2, tl_online_help(''Topic'',''TL_Sum''),else, web([''jar:file:///'',matlabroot,''/help/toolbox/simulink/help.jar!/slref/' lower(get_param(gcbh,'Blocktype')) '.html''], ''-helpbrowser''),end'])
      mask Display: plot([-0.05, 1.05, NaN, -0.05, 1.05],[.01, .01, NaN, .99, .99])
  Merge : Merge  RequirementInfo={} %GIDa_a87ba109_53e6_4c2e_ac2e_5fa8c249b378  Inputs=3  InitialOutput=0  mask(TL_Merge){data={'date',735951.66846518521}}
      settings: CopyFcn=if exist('tl_reset_reviewflag','file')==2,tl_reset_reviewflag(gcbh);end  DeleteFcn=if exist('delete_tlblock','file')==2,delete_tlblock(gcbh);end  NameChangeFcn=if exist('rename_tlblock','file')==2,rename_tlblock(gcbh);end  OpenFcn=if exist('tl_open_blockdlg','file')==2,tl_open_blockdlg(gcbh);else,open_system(gcbh,'parameter');end
      mask Help: eval(['if exist(''tl_online_help'',''file'') == 2, tl_online_help(''Topic'',''TL_Merge''),else, web([''jar:file:///'',matlabroot,''/help/toolbox/simulink/help.jar!/slref/' lower(get_param(gcbh,'Blocktype')) '.html''], ''-helpbrowser''),end'])
      mask Display: plot([-0.05, 1.05, NaN, -0.05, 1.05],[.01, .01, NaN, .99, .99])
  New Step : LIB_TF_G_12_StepControl/TF_G_12_ManageEndingStep/New Step  data={'output',{'variable','Internal_Interfaces/Enumerated_values/Step_Validity/KE_NEW_STEP'},'date',735951.6684861806}
  Relational Operator : RelationalOperator  RequirementInfo={} %GIDa_5e46c621_ae8a_4a36_9e39_bd975043b316  Operator=~=  OutDataTypeStr=boolean  mask(TL_RelationalOperator){data={'date',735951.66846481478}}
      settings: DeleteFcn=if exist('delete_tlblock','file')==2,delete_tlblock(gcbh);end  NameChangeFcn=if exist('rename_tlblock','file')==2,rename_tlblock(gcbh);end  OpenFcn=if exist('tl_open_blockdlg','file')==2,tl_open_blockdlg(gcbh);else,open_system(gcbh,'parameter');end
      mask Help: eval(['if exist(''tl_online_help'',''file'') == 2, tl_online_help(''Topic'',''TL_RelationalOperator''),else, web([''jar:file:///'',matlabroot,''/help/toolbox/simulink/help.jar!/slref/' lower(get_param(gcbh,'Blocktype')) '.html''], ''-helpbrowser''),end'])
      mask Display: plot([-0.05, 1.05, NaN, -0.05, 1.05],[.01, .01, NaN, .99, .99])
  Relational Operator2 : RelationalOperator  Operator===  OutDataTypeStr=boolean  mask(TL_RelationalOperator){data={'date',735951.6684852083}}
      settings: DeleteFcn=if exist('delete_tlblock','file')==2,delete_tlblock(gcbh);end  NameChangeFcn=if exist('rename_tlblock','file')==2,rename_tlblock(gcbh);end  OpenFcn=if exist('tl_open_blockdlg','file')==2,tl_open_blockdlg(gcbh);else,open_system(gcbh,'parameter');end
      mask Help: eval(['if exist(''tl_online_help'',''file'') == 2, tl_online_help(''Topic'',''TL_RelationalOperator''),else, web([''jar:file:///'',matlabroot,''/help/toolbox/simulink/help.jar!/slref/' lower(get_param(gcbh,'Blocktype')) '.html''], ''-helpbrowser''),end'])
      mask Display: plot([-0.05, 1.05, NaN, -0.05, 1.05],[.01, .01, NaN, .99, .99])
  Reset Counter 2 : Subsystem  RequirementInfo={} %GIDa_cdea1c29_55f4_4e4e_bec9_3f423aa2697f  TreatAsAtomicUnit=on
  Reset counter : Subsystem  RequirementInfo={} %GIDa_4d08dab9_6571_4c8a_bdd2_dad7dd1bc758  TreatAsAtomicUnit=on
  Unit Delay : UnitDelay  RequirementInfo={} %GIDa_f387a0d7_230e_404b_8167_cff67b785683  SampleTime=-1  mask(TL_UnitDelay){data={'output',{'type','Bool'},'state',{'type','Bool'},'date',735951.66846416669}}
      settings: CopyFcn=if exist('tl_reset_reviewflag','file')==2,tl_reset_reviewflag(gcbh);end  DeleteFcn=if exist('delete_tlblock','file')==2,delete_tlblock(gcbh);end  NameChangeFcn=if exist('rename_tlblock','file')==2,rename_tlblock(gcbh);end  OpenFcn=if exist('tl_open_blockdlg','file')==2,tl_open_blockdlg(gcbh);else,open_system(gcbh,'parameter');end
      mask Help: eval(['if exist(''tl_online_help'',''file'') == 2, tl_online_help(''Topic'',''TL_UnitDelay''),else, web([''jar:file:///'',matlabroot,''/help/toolbox/simulink/help.jar!/slref/' lower(get_param(gcbh,'Blocktype')) '.html''], ''-helpbrowser''),end'])
      mask Display: plot([-0.05, 1.05, NaN, -0.05, 1.05],[.01, .01, NaN, .99, .99])
  Unit Delay1 : UnitDelay  RequirementInfo={} %GIDa_92b2be4c_da1e_4587_a735_df4b9ebc41ea  SampleTime=-1  mask(TL_UnitDelay){data={'output',{'type','UInt8'},'state',{'type','UInt8'},'date',735951.66846363421}}
      settings: CopyFcn=if exist('tl_reset_reviewflag','file')==2,tl_reset_reviewflag(gcbh);end  DeleteFcn=if exist('delete_tlblock','file')==2,delete_tlblock(gcbh);end  NameChangeFcn=if exist('rename_tlblock','file')==2,rename_tlblock(gcbh);end  OpenFcn=if exist('tl_open_blockdlg','file')==2,tl_open_blockdlg(gcbh);else,open_system(gcbh,'parameter');end
      mask Help: eval(['if exist(''tl_online_help'',''file'') == 2, tl_online_help(''Topic'',''TL_UnitDelay''),else, web([''jar:file:///'',matlabroot,''/help/toolbox/simulink/help.jar!/slref/' lower(get_param(gcbh,'Blocktype')) '.html''], ''-helpbrowser''),end'])
      mask Display: plot([-0.05, 1.05, NaN, -0.05, 1.05],[.01, .01, NaN, .99, .99])
  bDecideToResetCounter : Logic  Operator=OR  AllPortsSameDT=off  OutDataTypeStr=boolean  mask(TL_LogicalOperator){data={'date',736308.63648153935}}
      settings: DeleteFcn=if exist('delete_tlblock','file')==2,delete_tlblock(gcbh);end  NameChangeFcn=if exist('rename_tlblock','file')==2,rename_tlblock(gcbh);end  OpenFcn=if exist('tl_open_blockdlg','file')==2,tl_open_blockdlg(gcbh);else,open_system(gcbh,'parameter');end
      mask Help: eval(['if exist(''tl_online_help'',''file'') == 2, tl_online_help(''Topic'',''TL_LogicalOperator''),else, web([''jar:file:///'',matlabroot,''/help/toolbox/simulink/help.jar!/slref/' lower(get_param(gcbh,'Blocktype')) '.html''], ''-helpbrowser''),end'])
      mask Display: plot([-0.05, 1.05, NaN, -0.05, 1.05],[.01, .01, NaN, .99, .99])
  u8Cnt : Outport  RequirementInfo={} %GIDa_aed58c49_27c6_4c05_bcd9_f288189eb3fe
  wires:
  u8Step/1 -> IncrementMotorBlockedCounter/1
  IncrementMotorBlockedCounter/1 -> u8Cnt/1, Unit Delay1/1
  bEdge/1 -> Relational Operator/1, Unit Delay/1, If/2
  Unit Delay/1 -> Relational Operator/2
  If/1 -> Reset counter/Action
  Relational Operator/1 -> bDecideToResetCounter/2
  Reset counter/1(Out1) -> Merge/1
  Merge/1 -> IncrementMotorBlockedCounter/2
  Unit Delay1/1 -> If Action Subsystem1/1(In1)
  If/2 -> If Action Subsystem1/Action
  If/3 -> Reset Counter 2/Action
  If Action Subsystem1/1(Out1) -> Merge/2
  Reset Counter 2/1(Out1) -> Merge/3
  New Step/1 -> Relational Operator2/1
  e_StepValidity/1 -> Relational Operator2/2
  Relational Operator2/1 -> bDecideToResetCounter/1
  bDecideToResetCounter/1 -> If/1

== system LIB_TF_G_12_StepControl/TF_G_12_ManageEndingStep/Step execution in progress/ManageMotorBlocked (Motor OverCurrent)/Motor Blocked Opt Activated/If Action Subsystem1/Integrator with u8 saturation/If Action Subsystem1 ==
  In1 : Inport  RequirementInfo={} %GIDa_92bdd9db_243b_4036_a296_b59854dbdc33
  Action Port : ActionPort  RequirementInfo={} %GIDa_3fb3a89d_f722_49a0_8458_67c5afdb1569
  Out1 : Outport  RequirementInfo={} %GIDa_bdaeb674_dd43_4362_8607_d7704cb5a332
  wires:
  In1/1 -> Out1/1

== system LIB_TF_G_12_StepControl/TF_G_12_ManageEndingStep/Step execution in progress/ManageMotorBlocked (Motor OverCurrent)/Motor Blocked Opt Activated/If Action Subsystem1/Integrator with u8 saturation/Reset Counter 2 ==
  Action Port : ActionPort  RequirementInfo={} %GIDa_a9d1cd47_cf0b_472a_b8af_80eeb1a6b757
  KU8_ZERO : Constant  RequirementInfo={} %GIDa_d5198ca9_62a3_45fa_973c_8a8c4ea2601b  Value=ddv('Common/KU8_ZERO')  OutDataTypeStr=uint8  SampleTime=-1  mask(TL_Constant){data={'output',{'variable','Common/KU8_ZERO'},'date',735951.66846556717}}
      settings: CopyFcn=if exist('tl_reset_reviewflag','file')==2,tl_reset_reviewflag(gcbh);end  DeleteFcn=if exist('delete_tlblock','file')==2,delete_tlblock(gcbh);end  NameChangeFcn=if exist('rename_tlblock','file')==2,rename_tlblock(gcbh);end  OpenFcn=if exist('tl_open_blockdlg','file')==2,tl_open_blockdlg(gcbh);else,open_system(gcbh,'parameter');end
      mask Help: eval(['if exist(''tl_online_help'',''file'') == 2, tl_online_help(''Topic'',''TL_Constant''),else, web([''jar:file:///'',matlabroot,''/help/toolbox/simulink/help.jar!/slref/' lower(get_param(gcbh,'Blocktype')) '.html''], ''-helpbrowser''),end'])
      mask Display: plot([-0.05, 1.05, NaN, -0.05, 1.05],[.01, .01, NaN, .99, .99])
  Out1 : Outport  RequirementInfo={} %GIDa_3d9f5f7e_d944_433f_9208_26f84a0ab520  InitialOutput=0
  wires:
  KU8_ZERO/1 -> Out1/1

== system LIB_TF_G_12_StepControl/TF_G_12_ManageEndingStep/Step execution in progress/ManageMotorBlocked (Motor OverCurrent)/Motor Blocked Opt Activated/If Action Subsystem1/Integrator with u8 saturation/Reset counter ==
  Action Port : ActionPort  RequirementInfo={} %GIDa_8f8c5ad8_e8c9_4108_b155_dc06b6872102
  KU8_ZERO : Constant  RequirementInfo={} %GIDa_59e5a77c_299a_4554_bd9b_ae4cab18b3c9  Value=ddv('Common/KU8_ZERO')  OutDataTypeStr=uint8  SampleTime=-1  mask(TL_Constant){data={'output',{'variable','Common/KU8_ZERO'},'date',735951.66846593749}}
      settings: CopyFcn=if exist('tl_reset_reviewflag','file')==2,tl_reset_reviewflag(gcbh);end  DeleteFcn=if exist('delete_tlblock','file')==2,delete_tlblock(gcbh);end  NameChangeFcn=if exist('rename_tlblock','file')==2,rename_tlblock(gcbh);end  OpenFcn=if exist('tl_open_blockdlg','file')==2,tl_open_blockdlg(gcbh);else,open_system(gcbh,'parameter');end
      mask Help: eval(['if exist(''tl_online_help'',''file'') == 2, tl_online_help(''Topic'',''TL_Constant''),else, web([''jar:file:///'',matlabroot,''/help/toolbox/simulink/help.jar!/slref/' lower(get_param(gcbh,'Blocktype')) '.html''], ''-helpbrowser''),end'])
      mask Display: plot([-0.05, 1.05, NaN, -0.05, 1.05],[.01, .01, NaN, .99, .99])
  Out1 : Outport  RequirementInfo={} %GIDa_12563ecb_1b8a_420c_b403_e93564dbdfdd  InitialOutput=0
  wires:
  KU8_ZERO/1 -> Out1/1
